simulink model "task2_tf"  (R2024a)
settings: Solver=VariableStepAuto  StartTime=0.0  StopTime=10.0  RelTol=1e-3
settings Model: Creator=kit  LastModifiedBy=kit

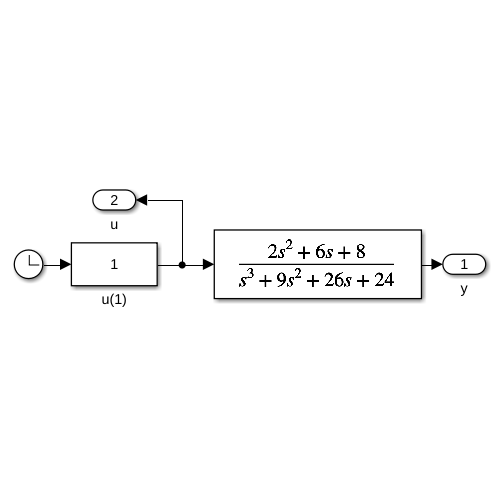
[thumbnail: Simulink's stored preview of the top-level diagram]
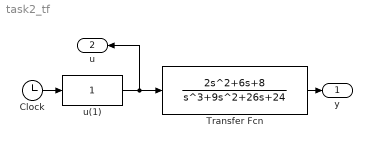
== system task2_tf ==
  Clock : Clock
  Transfer Fcn : TransferFcn  Numerator=[2 6 8]  Denominator=[1 9 26 24]
  u(1) : Fcn  Expr=1
  y : Outport
  u : Outport  Port=2
  wires:
  Clock/1 -> u(1)/1
  u(1)/1 -> u/1, Transfer Fcn/1
  Transfer Fcn/1 -> y/1
